simulink model "psbgui"  (Simulink 6.0)
settings: Solver=ode15s  SolverMode=SingleTasking  StartTime=0.0  StopTime=0.05  RelTol=1e-4
InitFcn:
  | powericon('psbinitsys',bdroot);
libraries: powerlib2 x30
settings Model: Creator=patrice  LastModifiedBy=batserve  ExtModeTrigMode=oneshot  ExtModeArmWhenConnect=off  ExtModeAutoUpdateStatusClock=off
settings DataIOCC: ExternalInput=[]  LimitDataPoints=off  SaveOutput=off  SignalLoggingName=sigsOut
settings OptimizationCC: BlockReduction=off  BooleanDataType=off
settings DebuggingCC: AlgebraicLoopMsg=none  SolverPrmCheckMsg=none
settings HardwareCC: TargetUnknown=on
settings RTWCC: TemplateMakefile=grt_unix.tmf

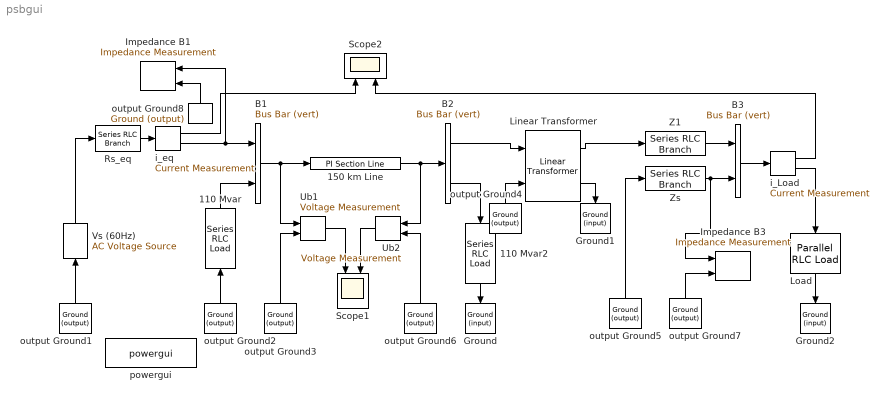
== system psbgui ==
  110 Mvar : powerlib2/Elements/Series RLC Load  Tag=PoWeRsYsTeMbLoCk  Orientation=up  a=735000/sqrt(3)  b=60  c=110e6/300  d=110e6  e=0  mesure=None  PSBOutputType=1
  110 Mvar2 : powerlib2/Elements/Series RLC Load  Tag=PoWeRsYsTeMbLoCk  Orientation=down  a=735000/sqrt(3)  b=60  c=110e6/300  d=110e6  e=0  mesure=None  PSBOutputType=1
  150 km Line : powerlib2/Elements/PI Section Line  Tag=PoWeRsYsTeMbLoCk  f=60  a=0.011  b=0.8674e-03  c=13.41e-09  d=150  e=2  mesure=None  PSBOutputType=1
  B1 : powerlib2/Connectors/Bus Bar (vert)  Tag=PoWeRsYsTeMbLoCk  entrees=2  sorties=1  PSBOutputType=11111111111111111111111111111111111111111111111111111111111111111111111111111111111111111
  B2 : powerlib2/Connectors/Bus Bar (vert)  Tag=PoWeRsYsTeMbLoCk  entrees=1  sorties=2  PSBOutputType=11111111111111111111111111111111111111111111111111111111111111111111111111111111111111111
  B3 : powerlib2/Connectors/Bus Bar (vert)  Tag=PoWeRsYsTeMbLoCk  entrees=2  sorties=1  PSBOutputType=11111111111111111111111111111111111111111111111111111111111111111111111111111111111111111
  Ground : powerlib2/Connectors/Ground (input)  Tag=PoWeRsYsTeMbLoCk  Orientation=down
  Ground1 : powerlib2/Connectors/Ground (input)  Tag=PoWeRsYsTeMbLoCk  Orientation=down
  Ground2 : powerlib2/Connectors/Ground (input)  Tag=PoWeRsYsTeMbLoCk  Orientation=down
  Impedance B1 : powerlib2/Measurements/Impedance Measurement  Tag=PoWeRsYsTeMbLoCk  Orientation=left  kz=1
  Impedance B3 : powerlib2/Measurements/Impedance Measurement  Tag=PoWeRsYsTeMbLoCk  kz=1
  Linear Transformer : powerlib2/Elements/Linear Transformer  Tag=PoWeRsYsTeMbLoCk  a=[750e6/3,60]  b=[735000/sqrt(3), 0.001 ,0.15]  c=[315000/sqrt(3), 0.001,0]  w3check=off  d=[315000/sqrt(3), 0.001,0]  e=[500 500]  mesure=None  PSBOutputType=1111
  Load : powerlib2/Elements/Parallel RLC Load  Tag=PoWeRsYsTeMbLoCk  Orientation=down  a=315000/sqrt(3)  b=60  c=200e6  d=0  e=50e6  mesure=None  PSBOutputType=1
  Rs_eq : powerlib2/Elements/Series RLC Branch  Tag=PoWeRsYsTeMbLoCk  a=2  b=0  c=inf  mesure=None  PSBOutputType=1
  Scope1 : Scope  NumInputPorts=2
      settings: Orientation=down  TimeRange=0.05  YMin=-1000000~-1000000  YMax=1000000~1000000
  Scope2 : Scope  NumInputPorts=2
      settings: Orientation=up  TimeRange=0.05  YMin=-1000~-2000  YMax=3000~2000
  Ub1 : powerlib2/Measurements/Voltage Measurement  Tag=PoWeRsYsTeMmEaSuReMeNt  PhasorSimulation=off  OutputType=Magnitude  PSBOutputType=0  PSBequivalent=0
  Ub2 : powerlib2/Measurements/Voltage Measurement  Tag=PoWeRsYsTeMmEaSuReMeNt  Orientation=left  PhasorSimulation=off  OutputType=Magnitude  PSBOutputType=0  PSBequivalent=0
  Vs (60Hz) : powerlib2/Electrical Sources/AC Voltage Source  Tag=PoWeRsYsTeMbLoCk  Orientation=up  A=735000/sqrt(3)*sqrt(2)  P=0  F=60  stime=0  mesure=None  PSBOutputType=1
  Z1 : powerlib2/Elements/Series RLC Branch  Tag=PoWeRsYsTeMbLoCk  a=0.734  b=0.02085  c=inf  mesure=None  PSBOutputType=1
  Zs : powerlib2/Elements/Series RLC Branch  Tag=PoWeRsYsTeMbLoCk  a=11.0  b=0.2925  c=inf  mesure=None  PSBOutputType=1
  i_Load : powerlib2/Measurements/Current Measurement  Tag=PoWeRsYsTeMmEaSuReMeNt  PhasorSimulation=off  OutputType=Magnitude  PSBOutputType=01  PSBequivalent=0
  i_eq : powerlib2/Measurements/Current Measurement  Tag=PoWeRsYsTeMmEaSuReMeNt  PhasorSimulation=off  OutputType=Magnitude  PSBOutputType=01  PSBequivalent=0
  output Ground{1..8} (8 alike) : powerlib2/Connectors/Ground (output)  Tag=PoWeRsYsTeMbLoCk  Orientation=up  PSBOutputType=1
  powergui : powerlib2/powergui  Frange=logspace(0,3,50)  Ylog=off  Xlog=off  save=off  variable=ZData  ZoomFFT=on  StartTime=0.0  cycles=2  DisplayStyle=off  fundamental=60  FreqAxis=off  MaxFrequency=1000  frequencyindice=1  frequencyindicesteady=1  RmsSteady=1  display=off  Ts=0  methode=off  frequency=60  echomessages=off
  wires:
  output Ground1/1 -> Vs (60Hz)/1
  Vs (60Hz)/1 -> Rs_eq/1
  output Ground2/1 -> 110 Mvar/1
  110 Mvar/1 -> B1/2
  i_eq/1 -> Scope2/1
  Rs_eq/1 -> i_eq/1
  B2/2 -> 110 Mvar2/1
  110 Mvar2/1 -> Ground/1
  B1/1 -> 150 km Line/1, Ub1/1
  output Ground3/1 -> Ub1/2
  150 km Line/1 -> B2/1, Ub2/1
  output Ground6/1 -> Ub2/2
  Ub1/1 -> Scope1/1
  Ub2/1 -> Scope1/2
  Linear Transformer/2 -> Ground1/1
  output Ground4/1 -> Linear Transformer/2
  B2/1 -> Linear Transformer/1
  Z1/1 -> B3/1
  Load/1 -> Ground2/1
  i_Load/2 -> Load/1
  i_Load/1 -> Scope2/2
  output Ground5/1 -> Zs/1
  Linear Transformer/1 -> Z1/1
  output Ground7/1 -> Impedance B3/2
  B3/1 -> i_Load/1
  Zs/1 -> B3/2, Impedance B3/1
  i_eq/2 -> B1/1, Impedance B1/1
  output Ground8/1 -> Impedance B1/2
